simulink model "k1vissr3p"  (Simulink 8.8)
settings: Solver=ode45  StartTime=0.0  StopTime=10.0  RelTol=1e-3  EnableMultiTasking=on
libraries: cdsIPCx x13, cdsCDI64 x3, cdsCDO64 x3, PAYLOAD_MASTER x3, dac x2, cdsAdcx0 x1, cdsParameters x1
settings Model: SuppressorTable=22 serialization::archive 11 0 3 0 0 0 11 0  Creator=controls  LastModifiedBy=controls
settings DataIOCC: SignalLoggingSaveFormat=Dataset
settings DebuggingCC: UnderspecifiedInitializationDetection=Simplified  MergeDetectMultiDrivingBlocksExec=error  FcnCallInpInsideContextMsg=error  AllowSymbolicDim=off  StateNameClashWarn=none
settings GRTTargetCC: CombineOutputUpdateFcns=on  GRTInterface=off

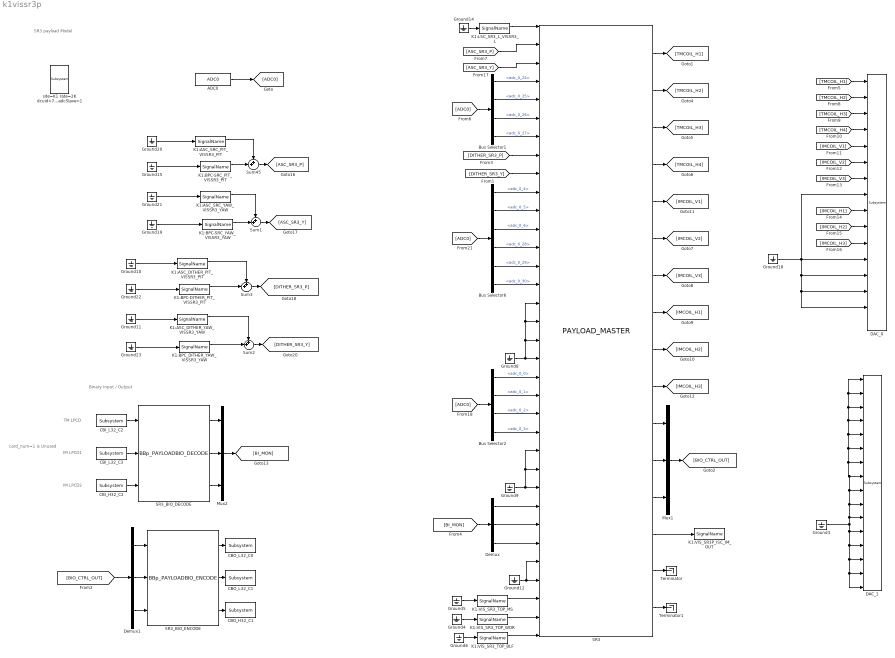
== system k1vissr3p ==
  note: SR3 payload Model
  note: Binary Input / Output
  note: card_num=1 is Unused
  note: TM LPCD
  note: IM LPCD1
  note: IM LPCD2
  ADC0 : cdsAdcx0/ADC0  Tag=cdsAdc  Description=|
      | type-GSC_16AI64SSA
      | card_num=0
      settings: AttributesFormatString=%<Description>\n%<Tag>
  Bus Selector1 : BusSelector  Description=ADC Selector  OutputSignals=adc_0_24,adc_0_25,adc_0_26,adc_0_27
      settings: AttributesFormatString=%<Description>
  Bus Selector2 : BusSelector  Description=ADC Selector  OutputSignals=adc_0_0,adc_0_1,adc_0_2,adc_0_3
      settings: AttributesFormatString=%<Description>
  Bus Selector6 : BusSelector  Description=ADC Selector  OutputSignals=adc_0_4,adc_0_5,adc_0_6,adc_0_28,adc_0_29,adc_0_30
      settings: AttributesFormatString=%<Description>
  CBI_H32_C2 : cdsCDI64/Subsystem  Tag=cdsCDI64  Description=card_num=3
      settings: AttributesFormatString=%<Tag>\n%<Description>
  CBI_L32_C2 : cdsCDI64/Subsystem  Tag=cdsCDI64  Description=card_num=0
      settings: AttributesFormatString=%<Tag>\n%<Description>
  CBI_L32_C3 : cdsCDI64/Subsystem  Tag=cdsCDI64  Description=card_num=2
      settings: AttributesFormatString=%<Tag>\n%<Description>
  CBO_H32_C1 : cdsCDO64/Subsystem  Tag=cdsCDO64  Description=card_num=3
      settings: AttributesFormatString=%<Tag>\n%<Description>
  CBO_L32_C0 : cdsCDO64/Subsystem  Tag=cdsCDO64  Description=card_num=0
      settings: AttributesFormatString=%<Tag>\n%<Description>
  CBO_L32_C1 : cdsCDO64/Subsystem  Tag=cdsCDO64  Description=card_num=2
      settings: AttributesFormatString=%<Tag>\n%<Description>
  DAC_0 : dac/Subsystem  Description=|
      | type=GSC_16AO16,
      | card_num=0
      settings: AttributesFormatString=%<Description>
  DAC_1 : dac/Subsystem  Description=|
      | type=GSC_16AO16,
      | card_num=1
      settings: AttributesFormatString=%<Description>
  Demux : Demux  Outputs=3
  Demux1 : Demux  Outputs=3
  Ground{3..6,8..12,14..15,18..23} (17 alike) : Ground
  K1:ASC_DITHER_PIT_VISSR3_PIT : cdsIPCx/SignalName  Tag=cdsIPCx_PCIE  Description=Inter-Process Communication via PCI Express network.
      settings: AttributesFormatString=%<Tag>
  K1:ASC_DITHER_YAW_VISSR3_YAW : cdsIPCx/SignalName  Tag=cdsIPCx_PCIE  Description=Inter-Process Communication via PCI Express network.
      settings: AttributesFormatString=%<Tag>
  K1:ASC_SRC_PIT_VISSR3_PIT : cdsIPCx/SignalName  Tag=cdsIPCx_PCIE  Description=Inter-Process Communication via PCI Express network.
      settings: AttributesFormatString=%<Tag>
  K1:ASC_SRC_YAW_VISSR3_YAW : cdsIPCx/SignalName  Tag=cdsIPCx_PCIE  Description=Inter-Process Communication via PCI Express network.
      settings: AttributesFormatString=%<Tag>
  K1:BPC-DITHER_PIT_VISSR3_PIT : cdsIPCx/SignalName  Tag=cdsIPCx_PCIE  Description=Inter-Process Communication via PCI Express network.
      settings: AttributesFormatString=%<Tag>
  K1:BPC-SRC_PIT_VISSR3_PIT : cdsIPCx/SignalName  Tag=cdsIPCx_PCIE  Description=Inter-Process Communication via PCI Express network.
      settings: AttributesFormatString=%<Tag>
  K1:BPC-SRC_YAW_VISSR3_YAW : cdsIPCx/SignalName  Tag=cdsIPCx_PCIE  Description=Inter-Process Communication via PCI Express network.
      settings: AttributesFormatString=%<Tag>
  K1:BPC_DITHER_YAW_VISSR3_YAW : cdsIPCx/SignalName  Tag=cdsIPCx_PCIE  Description=Inter-Process Communication via PCI Express network.
      settings: AttributesFormatString=%<Tag>
  K1:LSC_SR3_L_VISSR3_L : cdsIPCx/SignalName  Tag=cdsIPCx_PCIE  Description=Inter-Process Communication via PCI Express network.
      settings: AttributesFormatString=%<Tag>
  K1:VIS_SR3P_ISC_IM_OUT : cdsIPCx/SignalName  Tag=cdsIPCx_SHMEM  Description=Inter-Process Communication via Shared memory.
      settings: AttributesFormatString=%<Tag>
  K1:VIS_SR3_TOP_BLF : cdsIPCx/SignalName  Tag=cdsIPCx_SHMEM  Description=Inter-Process Communication via Shared memory.
      settings: AttributesFormatString=%<Tag>
  K1:VIS_SR3_TOP_MS : cdsIPCx/SignalName  Tag=cdsIPCx_SHMEM  Description=Inter-Process Communication via Shared memory.
      settings: AttributesFormatString=%<Tag>
  K1:VIS_SR3_TOP_WDR : cdsIPCx/SignalName  Tag=cdsIPCx_SHMEM  Description=Inter-Process Communication via Shared memory.
      settings: AttributesFormatString=%<Tag>
  Mux1 : Mux  Inputs=3
  Mux2 : Mux  Inputs=3
  SR3 : PAYLOAD_MASTER/PAYLOAD_MASTER  Description=This is for Type-B and Bp payloads.
      settings: AttributesFormatString=%<Description>
  SR3_BIO_DECODE : PAYLOAD_MASTER/BBp_PAYLOADBIO_DECODE
  SR3_BIO_ENCODE : PAYLOAD_MASTER/BBp_PAYLOADBIO_ENCODE
  Sum{1..3,45} (4 alike) : Sum  Inputs=++|
  Terminator : Terminator
  Terminator1 : Terminator
  site=K1 rate=2K dcuid=71 host=k1sr3 specific_cpu=3 adcSlave=1 : cdsParameters/Subsystem  Tag=cdsParameters  Description=|
      | Purpose:                                                                                                                                                                                                                                
      | Provide system parameters to the FE code generator to properly configure the generated EPICS names, rep rate of the FE controller, and the Data Acquisition node ID for proper storage of data from this FE controller.                 
      |                                                                                                                                                                                                                                         
      | Useage:                                                                                                                                                                                                                                 
      | The part NAME field is used to identify the FE parameters. It must be of the form:                                                                                                                                                      
      | site=                                                                                                                                                                                                                                   
      | rate=                                                                                                                                                                                                                                   
      | dcuid=                                                                                                                                                                                                                                  
      |                                                                                                                                                                                                                                         
      | Where:                                                                                                                                                                                                                                  
      | site= argument may be H1, H2, L1, M1, G1, either as a single argument or multiple, for example site=H1,H2. These are the only names allowed. These will become the first two characters of all EPICS and signal names (for example G1:).
      |                                                                                                                                                                                                                                         
      | rate= may be 2K, 16K, 32K, or 64K                                                                                                                                                                                                       
      |                                                                                                                                                                                                                                         
      | dcuid= is site specific ie it must be unique at each site.
      settings: AttributesFormatString=%<Tag>
  wires:
  ADC0/1 -> [ADC0]
  [ADC0] -> Bus Selector6/1
  Ground18/1 -> DAC_0/12, DAC_0/13, DAC_0/14, DAC_0/15, DAC_0/8
  [TMCOIL_H2] -> DAC_0/2
  [TMCOIL_H3] -> DAC_0/3
  [TMCOIL_H1] -> DAC_0/1
  [TMCOIL_H4] -> DAC_0/4
  [IMCOIL_V1] -> DAC_0/5
  [IMCOIL_V2] -> DAC_0/6
  [IMCOIL_V3] -> DAC_0/7
  [IMCOIL_H3] -> DAC_0/11
  [IMCOIL_H2] -> DAC_0/10
  [IMCOIL_H1] -> DAC_0/9
  Mux1/1 -> [BIO_CTRL_OUT]
  [BI_MON] -> Demux/1
  Ground4/1 -> K1:VIS_SR3_TOP_WDR/1
  Ground5/1 -> K1:VIS_SR3_TOP_MS/1
  Ground3/1 -> DAC_1/13, DAC_1/14, DAC_1/15, DAC_1/16, DAC_1/12, DAC_1/7, DAC_1/6, DAC_1/5, DAC_1/1, DAC_1/2, DAC_1/3, DAC_1/4, DAC_1/8, DAC_1/9, DAC_1/10, DAC_1/11
  CBI_L32_C3/1 -> SR3_BIO_DECODE/2
  CBI_H32_C2/1 -> SR3_BIO_DECODE/3
  SR3_BIO_DECODE/2 -> Mux2/2
  SR3_BIO_DECODE/3 -> Mux2/3
  SR3_BIO_DECODE/1 -> Mux2/1
  Mux2/1 -> [BI_MON]
  CBI_L32_C2/1 -> SR3_BIO_DECODE/1
  SR3_BIO_ENCODE/1 -> CBO_L32_C0/1
  SR3_BIO_ENCODE/3 -> CBO_H32_C1/1
  SR3_BIO_ENCODE/2 -> CBO_L32_C1/1
  Demux1/2 -> SR3_BIO_ENCODE/2
  Demux1/3 -> SR3_BIO_ENCODE/3
  Demux1/1 -> SR3_BIO_ENCODE/1
  [BIO_CTRL_OUT] -> Demux1/1
  Ground6/1 -> K1:VIS_SR3_TOP_BLF/1
  Ground14/1 -> K1:LSC_SR3_L_VISSR3_L/1
  Sum45/1 -> [ASC_SR3_P]
  K1:ASC_SRC_PIT_VISSR3_PIT/1 -> Sum45/1
  Sum1/1 -> [ASC_SR3_Y]
  K1:ASC_SRC_YAW_VISSR3_YAW/1 -> Sum1/1
  K1:BPC-SRC_YAW_VISSR3_YAW/1 -> Sum1/2
  K1:BPC-SRC_PIT_VISSR3_PIT/1 -> Sum45/2
  Sum3/1 -> [DITHER_SR3_P]
  K1:ASC_DITHER_PIT_VISSR3_PIT/1 -> Sum3/1
  Sum2/1 -> [DITHER_SR3_Y]
  K1:ASC_DITHER_YAW_VISSR3_YAW/1 -> Sum2/1
  K1:BPC-DITHER_PIT_VISSR3_PIT/1 -> Sum3/2
  Ground22/1 -> K1:BPC-DITHER_PIT_VISSR3_PIT/1
  Ground23/1 -> K1:BPC_DITHER_YAW_VISSR3_YAW/1
  K1:BPC_DITHER_YAW_VISSR3_YAW/1 -> Sum2/2
  Ground20/1 -> K1:ASC_SRC_PIT_VISSR3_PIT/1
  Ground21/1 -> K1:ASC_SRC_YAW_VISSR3_YAW/1
  Ground10/1 -> K1:ASC_DITHER_PIT_VISSR3_PIT/1
  Ground11/1 -> K1:ASC_DITHER_YAW_VISSR3_YAW/1
  Ground15/1 -> K1:BPC-SRC_PIT_VISSR3_PIT/1
  Ground19/1 -> K1:BPC-SRC_YAW_VISSR3_YAW/1
  SR3/7 -> [IMCOIL_V3]
  SR3/6 -> [IMCOIL_V2]
  SR3/5 -> [IMCOIL_V1]
  SR3/8 -> [IMCOIL_H1]
  SR3/9 -> [IMCOIL_H2]
  SR3/10 -> [IMCOIL_H3]
  SR3/4 -> [TMCOIL_H4]
  SR3/3 -> [TMCOIL_H3]
  SR3/2 -> [TMCOIL_H2]
  SR3/1 -> [TMCOIL_H1]
  SR3/12 -> Mux1/2
  SR3/11 -> Mux1/1
  SR3/13 -> Mux1/3
  SR3/14 -> K1:VIS_SR3P_ISC_IM_OUT/1
  SR3/15 -> Terminator/1
  SR3/16 -> Terminator1/1
  K1:LSC_SR3_L_VISSR3_L/1 -> SR3/1
  [ASC_SR3_P] -> SR3/2
  [ASC_SR3_Y] -> SR3/3
  [ADC0] -> Bus Selector1/1
  Bus Selector1/1 -> SR3/4  "<adc_0_24>"
  Bus Selector1/2 -> SR3/5  "<adc_0_25>"
  Bus Selector1/3 -> SR3/6  "<adc_0_26>"
  Bus Selector1/4 -> SR3/7  "<adc_0_27>"
  [DITHER_SR3_P] -> SR3/8
  [DITHER_SR3_Y] -> SR3/9
  Bus Selector6/6 -> SR3/15  "<adc_0_30>"
  Bus Selector6/5 -> SR3/14  "<adc_0_29>"
  Bus Selector6/4 -> SR3/13  "<adc_0_28>"
  Bus Selector6/3 -> SR3/12  "<adc_0_6>"
  Bus Selector6/2 -> SR3/11  "<adc_0_5>"
  Bus Selector6/1 -> SR3/10  "<adc_0_4>"
  Ground8/1 -> SR3/18, SR3/17, SR3/16, SR3/19
  [ADC0] -> Bus Selector2/1
  Bus Selector2/1 -> SR3/20  "<adc_0_0>"
  Bus Selector2/2 -> SR3/21  "<adc_0_1>"
  Bus Selector2/3 -> SR3/22  "<adc_0_2>"
  Bus Selector2/4 -> SR3/23  "<adc_0_3>"
  Ground9/1 -> SR3/25, SR3/24, SR3/26
  Demux/1 -> SR3/27
  Demux/2 -> SR3/28
  Demux/3 -> SR3/29
  Ground12/1 -> SR3/30, SR3/31
  K1:VIS_SR3_TOP_MS/1 -> SR3/32
  K1:VIS_SR3_TOP_WDR/1 -> SR3/33
  K1:VIS_SR3_TOP_BLF/1 -> SR3/34
